simulink model "Atividade6"  (R2017a)
settings: Solver=VariableStepAuto  StartTime=0.0  StopTime=10.0  RelTol=1e-3
settings Model: Creator=mariajulia  LastModifiedBy=mariajulia

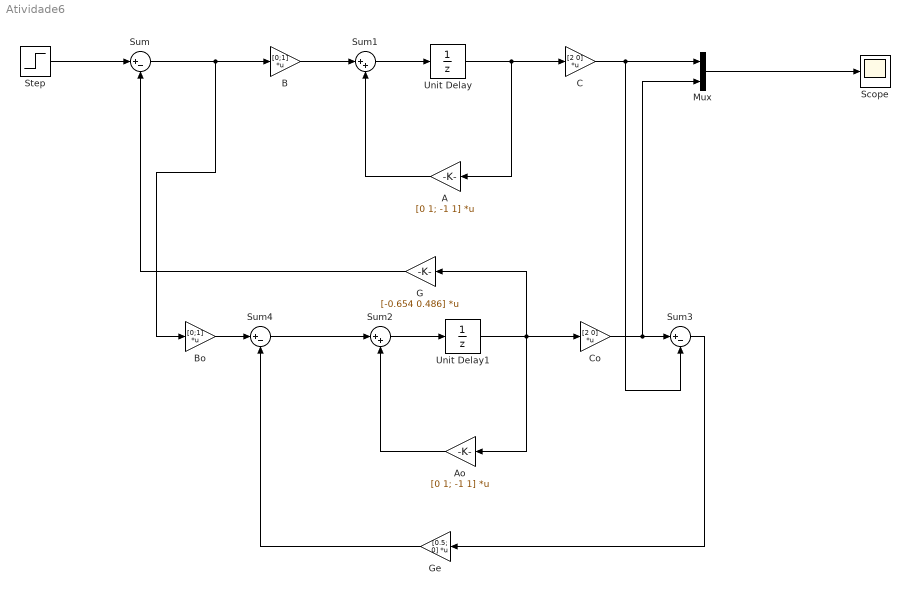
== system Atividade6 ==
  A : Gain  Gain=[0 1; -1 1]  Multiplication=Matrix(K*u)
  Ao : Gain  Gain=[0 1; -1 1]  Multiplication=Matrix(K*u)
  B : Gain  Gain=[0;1]  Multiplication=Matrix(K*u)
  Bo : Gain  Gain=[0;1]  Multiplication=Matrix(K*u)
  C : Gain  Gain=[2 0]  Multiplication=Matrix(K*u)
  Co : Gain  Gain=[2 0]  Multiplication=Matrix(K*u)
  G : Gain  Gain=[-0.654 0.486]  Multiplication=Matrix(K*u)
  Ge : Gain  Gain=[0.5; 0]  Multiplication=Matrix(K*u)
  Mux : Mux  Inputs=2
  Scope : Scope
  Step : Step  SampleTime=0
  Sum : Sum  Inputs=|+-
  Sum1 : Sum  Inputs=|++
  Sum2 : Sum  Inputs=|++
  Sum3 : Sum  Inputs=|+-
  Sum4 : Sum  Inputs=|+-
  Unit Delay : UnitDelay  InitialCondition=1  SampleTime=-1
  Unit Delay1 : UnitDelay  SampleTime=-1
  wires:
  Mux/1 -> Scope/1
  C/1 -> Sum3/2, Mux/1
  Unit Delay/1 -> A/1, C/1
  A/1 -> Sum1/2
  Sum1/1 -> Unit Delay/1
  B/1 -> Sum1/1
  G/1 -> Sum/2
  Step/1 -> Sum/1
  Unit Delay1/1 -> G/1, Ao/1, Co/1
  Ao/1 -> Sum2/2
  Sum2/1 -> Unit Delay1/1
  Co/1 -> Mux/2, Sum3/1
  Sum3/1 -> Ge/1
  Bo/1 -> Sum4/1
  Ge/1 -> Sum4/2
  Sum4/1 -> Sum2/1
  Sum/1 -> Bo/1, B/1
